simulink model "Multi_drones_final_results"  (R2021a)
settings: Solver=ode4  StartTime=0.0  StopTime=50  FixedStep=0.005  RelTol=1e-3
(part 4 of 7)

== system Multi_drones_final_results/Controller 4/Controller/Attitude controller/Sliding mode differentiator/Second-order derivative ==
  ang_d_dot : Inport
  t : Inport  Port=2
  First derivative : MATLAB Function  TreatAsAtomicUnit=on
  Memory : Memory  InitialCondition=[0;0;0]
  Memory1 : Memory
  Memory2 : Memory  InitialCondition=[0;0;0]
  ang_d_ddot : Outport
  wires:
  ang_d_dot/1 -> First derivative/1(ang_d_dot)
  First derivative/1(ang_d_ddot) -> Memory2/1
  t/1 -> First derivative/2(t)
  First derivative/3(loop_num) -> Memory1/1
  Memory1/1 -> First derivative/5("loop_num ")
  First derivative/2(ang_d_dot_prev) -> Memory/1
  Memory/1 -> First derivative/3("ang_d_dot_prev ")
  Memory2/1 -> First derivative/4("ang_d_ddot "), ang_d_ddot/1

== system Multi_drones_final_results/Controller 4/Controller/Position controller1/Position loop observer/Single Layer Neural network ==
  state : Inport
  esti_s : Inport  Port=2
  Neural network output : MATLAB Function  TreatAsAtomicUnit=on
  Update of neural weight : MATLAB Function  TreatAsAtomicUnit=on
  Weight initialisation : MATLAB Function  TreatAsAtomicUnit=on
  Weight update : Integrator  InitialConditionSource=external
  w_i : Outport
  wires:
  Update of neural weight/1(W_dot) -> Weight update/1
  esti_s/1 -> Update of neural weight/2(esti_s)
  state/1 -> Update of neural weight/1(phi_net), Neural network output/1(phi_net)
  Neural network output/1(w_i) -> w_i/1
  Weight initialisation/1(W_0) -> Weight update/2
  Weight update/1 -> Update of neural weight/3(W), Neural network output/2(W)

== system Multi_drones_final_results/Controller 5/Controller/Attitude controller/Attitude loop observer/Single Layer Neural network ==
  state : Inport
  esti_s : Inport  Port=2
  Neural network output : MATLAB Function  TreatAsAtomicUnit=on
  Update of neural weight : MATLAB Function  TreatAsAtomicUnit=on
  Weight initialisation : MATLAB Function  TreatAsAtomicUnit=on
  Weight update : Integrator  InitialConditionSource=external
  w_i : Outport
  wires:
  Update of neural weight/1(W_dot) -> Weight update/1
  esti_s/1 -> Update of neural weight/2(esti_s)
  state/1 -> Update of neural weight/1(phi_net), Neural network output/1(phi_net)
  Neural network output/1(w_i) -> w_i/1
  Weight initialisation/1(W_0) -> Weight update/2
  Weight update/1 -> Update of neural weight/3(W), Neural network output/2(W)

== system Multi_drones_final_results/Controller 5/Controller/Attitude controller/Sliding mode differentiator/First-order derivative ==
  ang_d : Inport
  t : Inport  Port=2
  First derivative : MATLAB Function  TreatAsAtomicUnit=on
  Memory : Memory  InitialCondition=[0;0;0]
  Memory1 : Memory
  Memory2 : Memory  InitialCondition=[0;0;0]
  ang_d_dot : Outport
  wires:
  ang_d/1 -> First derivative/1(ang_d)
  First derivative/1(ang_d_dot) -> Memory2/1
  t/1 -> First derivative/2(t)
  First derivative/3(loop_num) -> Memory1/1
  Memory1/1 -> First derivative/5("loop_num ")
  First derivative/2(ang_d_prev) -> Memory/1
  Memory/1 -> First derivative/3("ang_d_prev ")
  Memory2/1 -> First derivative/4("ang_d_dot "), ang_d_dot/1

== system Multi_drones_final_results/Controller 5/Controller/Attitude controller/Sliding mode differentiator/Second-order derivative ==
  ang_d_dot : Inport
  t : Inport  Port=2
  First derivative : MATLAB Function  TreatAsAtomicUnit=on
  Memory : Memory  InitialCondition=[0;0;0]
  Memory1 : Memory
  Memory2 : Memory  InitialCondition=[0;0;0]
  ang_d_ddot : Outport
  wires:
  ang_d_dot/1 -> First derivative/1(ang_d_dot)
  First derivative/1(ang_d_ddot) -> Memory2/1
  t/1 -> First derivative/2(t)
  First derivative/3(loop_num) -> Memory1/1
  Memory1/1 -> First derivative/5("loop_num ")
  First derivative/2(ang_d_dot_prev) -> Memory/1
  Memory/1 -> First derivative/3("ang_d_dot_prev ")
  Memory2/1 -> First derivative/4("ang_d_ddot "), ang_d_ddot/1

== system Multi_drones_final_results/Controller 5/Controller/Position controller1/Position loop observer/Single Layer Neural network ==
  state : Inport
  esti_s : Inport  Port=2
  Neural network output : MATLAB Function  TreatAsAtomicUnit=on
  Update of neural weight : MATLAB Function  TreatAsAtomicUnit=on
  Weight initialisation : MATLAB Function  TreatAsAtomicUnit=on
  Weight update : Integrator  InitialConditionSource=external
  w_i : Outport
  wires:
  Update of neural weight/1(W_dot) -> Weight update/1
  esti_s/1 -> Update of neural weight/2(esti_s)
  state/1 -> Update of neural weight/1(phi_net), Neural network output/1(phi_net)
  Neural network output/1(w_i) -> w_i/1
  Weight initialisation/1(W_0) -> Weight update/2
  Weight update/1 -> Update of neural weight/3(W), Neural network output/2(W)

== system Multi_drones_final_results/Controller 6/Controller/Attitude controller/Attitude loop observer/Single Layer Neural network ==
  state : Inport
  esti_s : Inport  Port=2
  Neural network output : MATLAB Function  TreatAsAtomicUnit=on
  Update of neural weight : MATLAB Function  TreatAsAtomicUnit=on
  Weight initialisation : MATLAB Function  TreatAsAtomicUnit=on
  Weight update : Integrator  InitialConditionSource=external
  w_i : Outport
  wires:
  Update of neural weight/1(W_dot) -> Weight update/1
  esti_s/1 -> Update of neural weight/2(esti_s)
  state/1 -> Update of neural weight/1(phi_net), Neural network output/1(phi_net)
  Neural network output/1(w_i) -> w_i/1
  Weight initialisation/1(W_0) -> Weight update/2
  Weight update/1 -> Update of neural weight/3(W), Neural network output/2(W)

== system Multi_drones_final_results/Controller 6/Controller/Attitude controller/Sliding mode differentiator/First-order derivative ==
  ang_d : Inport
  t : Inport  Port=2
  First derivative : MATLAB Function  TreatAsAtomicUnit=on
  Memory : Memory  InitialCondition=[0;0;0]
  Memory1 : Memory
  Memory2 : Memory  InitialCondition=[0;0;0]
  ang_d_dot : Outport
  wires:
  ang_d/1 -> First derivative/1(ang_d)
  First derivative/1(ang_d_dot) -> Memory2/1
  t/1 -> First derivative/2(t)
  First derivative/3(loop_num) -> Memory1/1
  Memory1/1 -> First derivative/5("loop_num ")
  First derivative/2(ang_d_prev) -> Memory/1
  Memory/1 -> First derivative/3("ang_d_prev ")
  Memory2/1 -> First derivative/4("ang_d_dot "), ang_d_dot/1

== system Multi_drones_final_results/Controller 6/Controller/Attitude controller/Sliding mode differentiator/Second-order derivative ==
  ang_d_dot : Inport
  t : Inport  Port=2
  First derivative : MATLAB Function  TreatAsAtomicUnit=on
  Memory : Memory  InitialCondition=[0;0;0]
  Memory1 : Memory
  Memory2 : Memory  InitialCondition=[0;0;0]
  ang_d_ddot : Outport
  wires:
  ang_d_dot/1 -> First derivative/1(ang_d_dot)
  First derivative/1(ang_d_ddot) -> Memory2/1
  t/1 -> First derivative/2(t)
  First derivative/3(loop_num) -> Memory1/1
  Memory1/1 -> First derivative/5("loop_num ")
  First derivative/2(ang_d_dot_prev) -> Memory/1
  Memory/1 -> First derivative/3("ang_d_dot_prev ")
  Memory2/1 -> First derivative/4("ang_d_ddot "), ang_d_ddot/1

== system Multi_drones_final_results/Controller 6/Controller/Position controller1/Position loop observer/Single Layer Neural network ==
  state : Inport
  esti_s : Inport  Port=2
  Neural network output : MATLAB Function  TreatAsAtomicUnit=on
  Update of neural weight : MATLAB Function  TreatAsAtomicUnit=on
  Weight initialisation : MATLAB Function  TreatAsAtomicUnit=on
  Weight update : Integrator  InitialConditionSource=external
  w_i : Outport
  wires:
  Update of neural weight/1(W_dot) -> Weight update/1
  esti_s/1 -> Update of neural weight/2(esti_s)
  state/1 -> Update of neural weight/1(phi_net), Neural network output/1(phi_net)
  Neural network output/1(w_i) -> w_i/1
  Weight initialisation/1(W_0) -> Weight update/2
  Weight update/1 -> Update of neural weight/3(W), Neural network output/2(W)

== matlab function Multi_drones_final_results/Controller 3/Controller/Position controller1/Reference selection (Low) ==
  data: ref_x_p input; x_i_p_d output; v_i_p_d output; a_i_p_d output
function [x_i_p_d, v_i_p_d, a_i_p_d] = ref_selection(ref_x_p)

%% Description
% This function is built to separate the reference states

%% Reference dividing
x_i_p_d = ref_x_p(1:3);
v_i_p_d = ref_x_p(4:6);
a_i_p_d = ref_x_p(7:9);

end

== matlab function Multi_drones_final_results/Controller 3/Controller/Position controller1/State selection ==
  data: states_i input; x_i_p output; v_i_p output
function [x_i_p, v_i_p] = state_select(states_i)

%% Description
% This is the state selection model for the self-feedback
% x_ip, v_ip, x_ia, v_ia  -> x_i, v_i
% x_ip_d, v_ip_d, a_ip_d  -> ref_x_p
% psi_i_d  -> psi_i_d (not changing)

%% System states feedback
x_i = states_i(1:6);
v_i = states_i(7:12);

x_i_p = x_i(1:3);
v_i_p = v_i(1:3);

end

== matlab function Multi_drones_final_results/Controller 3/Controller/Position controller1/Virtual position controller ==
  data: w_hat_p input; s_i_p input; delta_x_p input; delta_v_p input; a_i_p_d input; u_i_p output
function u_i_p = virtual_position_control(w_hat_p, s_i_p, delta_x_p, delta_v_p, a_i_p_d)

%% Description
% This function generates the virtual control input for the position loop
% u_i_pos = [u_ix, u_iy, u_iz] is the control input for the position loop 

%% Parameters
lambda_i_p = 2;             %% You may want to change these values
k_i_p = 3;
c_i_p = 1;

g = 9.81;                   %% Gravity constant

%% Controller design
u_i_p = a_i_p_d - w_hat_p - lambda_i_p * delta_v_p - k_i_p * delta_x_p - c_i_p * s_i_p + [0;0;g];

end

== matlab function Multi_drones_final_results/Controller 3/Controller/Real control input ==
  data: tau_i output; u_i_a input; u_i output; T_id input
function [tau_i, u_i] = real_ctr(u_i_a, T_id)

%% This function is built to obtain the actual control input (motor force)
% The functions we have are:
% T_id = u_1 + u_2 + u_3 + u_4
% u_{i,4} = (R_i/J_i_x) * (- u_2 + u_4)
% u_{i,5} = (R_i/J_i_y) * (- u_1 + u_3)
% u_{i,6} = (upsilon_i/J_i_z) * (- u_1 + u_2 - u_3 + u_4)

%% Parameter selection        
R = [0.29, 0.31, 0.30, 0.32, 0.34, 0.33] ;                  %%%%%%%%%% Change if necc

J_x = [1.25,1.23,1.24,1.23,1.24,1.25];
J_y = [1.24,1.25,1.24,1.26,1.23,1.26];
J_z = [2.50,2.52,2.51,2.49,2.50,2.53];

upsilon = [51,52,49,51,48,53]/1000;       %% Reverse moment coefficent

%% Parameter selection
serial_num = 3;         %% -- Change the serial number here

R_i = R(serial_num);

J_i_x = J_x(serial_num);
J_i_y = J_y(serial_num);
J_i_z = J_z(serial_num);

upsilon_i = upsilon(serial_num);

g_i = [ 1,1,1,1;
        0, -R_i/J_i_x, 0, R_i/J_i_x;
       -R_i/J_i_y, 0, R_i/J_i_y, 0;
       -upsilon_i/J_i_z, upsilon_i/J_i_z, -upsilon_i/J_i_z, upsilon_i/J_i_z];

u_i = g_i^(-1) * [T_id;u_i_a];

tau_1 = - u_i(2) + u_i(4);
tau_2 = - u_i(1) + u_i(3); 
tau_3 = - u_i(1) + u_i(2) - u_i(3) + u_i(4); 

tau_i = [T_id; tau_1; tau_2; tau_3];


end

== matlab function Multi_drones_final_results/Controller 1/Controller/Position controller1/Position loop observer/MATLAB Function ==
  data: t input; w_hat_p output; w_hat_p input
function w_hat_p = smooth_intro(t, w_hat_p)

% if t<=2
%     w_hat_p = zeros(3,1);
% elseif (t>2 && t<=4)
%     w_hat_p = 0.25 * (t-2)^2 * w_hat_p;
% end

eta_2 = 4;
eta_3 = 2;

f = 1 - (exp(-eta_2 * (t - eta_3))/(1 + exp(-eta_2 * (t - eta_3))) );

w_hat_p = f * w_hat_p;

end

== matlab function Multi_drones_final_results/Controller 3/Controller/Reverse calculation/Reverse calculation ==
  data: psi_i_d input; u_i_p input; atti_ref output; T_i_d output; x_i_a input
function [atti_ref, T_i_d] = reverse_calculation(psi_i_d, u_i_p, x_i_a)

%% Basic parameters of the drone   
m = [0.88,0.90,0.91,0.90,0.89,0.92] + 1.2;             %%%%%%%%%% Change if necc

serial_num = 3;
m_i = m(serial_num);
g = 9.81; 

%% Decompose information

% u_i_p = u_i_p / m_i;

u_ix = u_i_p(1);
u_iy = u_i_p(2);
u_iz = u_i_p(3);
% u_iz = u_i_p(3) + g;

phi = x_i_a(1);
theta = x_i_a(2);
psi = x_i_a(3);


%% Reverse calculation
% T_i_d = m_i * sqrt(u_ix^2 + u_iy^2 + u_iz^2);
T_i_d = m_i * u_iz/(cos(phi) * cos(theta));
% T_i_d = m_i * (u_ix * (sin(theta) * cos(psi) * cos(phi) + sin(psi) * sin(phi)) + u_iy * (sin(theta) * sin(psi) * cos(phi) - cos(psi) * sin(phi)) + u_iz * cos(theta) * cos(phi) );

phi_i_d = asin( (u_ix * sin(psi_i_d) - u_iy * cos(psi_i_d) )/sqrt(u_ix^2 + u_iy^2 + u_iz^2) );
% phi_i_d = asin( (u_ix * sin(psi_i_d) - u_iy * cos(psi_i_d) )/T_i_d );
theta_i_d = atan( (u_ix * cos(psi_i_d) + u_iy *sin(psi_i_d) )/u_iz );

% Some possible restrictions
phi_i_d = sign(phi_i_d) * min(abs(phi_i_d), pi/3);
theta_i_d = sign(theta_i_d) * min(abs(theta_i_d), pi/3);

atti_ref = [phi_i_d; theta_i_d; psi_i_d];

end

== matlab function Multi_drones_final_results/Controller 3/Controller/Reverse calculation/State selection ==
  data: states_i input; x_i_a output
function x_i_a = state_selection(states_i)

x_i_a = states_i(4:6);

end

== matlab function Multi_drones_final_results/Controller 3/High-level system/Controller ==
  data: u_i output; delta_xi input; delta_vi input; s_i input; sat_dot input; a_di input
function u_i = low_control(delta_xi, delta_vi, s_i, sat_dot, a_di)

%% This is the controller design for each agent
%% Controller parameter
c_i = 1;
lambda_i = 2;
k_i = 1.5;

%% Nominal control input
u_i = a_di - c_i * s_i - lambda_i * diag(sat_dot) * delta_vi - k_i * delta_xi;

tau_i = 0.19;
psi = 0.01;

dimension = 3;

for i = 1 : dimension
   if abs(u_i(i)) <= tau_i
       continue;
   else
       u_i(i) = sign(u_i(i)) * (tau_i + psi*exp((tau_i - abs(u_i(i)))/psi ));
   end 
end

end

== matlab function Multi_drones_final_results/Controller 3/High-level system/Information subtracting ==
  data: L input; info_commu input; bar_delta input; delta_xi output; delta_vi output; s_i output; sat_dot output
function [delta_xi, delta_vi, s_i, sat_dot]=info_subtracting(L, info_commu, bar_delta)

%% This function is built to subtract the useful information for the controller design

% info_commu is in the format of [x_1,v_1,....,x_N,v_N]
% info_control is in the format of [delta_xi, delta_vi, a_di, w_i_hat]

dimension = 3;
lambda = 2;
serial_num = 3;

L_i = L(serial_num,:);

% For multiple system test: info_commu

x_sub = kron(kron(L_i,[1,0]),eye(dimension));
v_sub = kron(kron(L_i,[0,1]),eye(dimension));

e_xi = x_sub * info_commu;
e_vi = v_sub * info_commu;

% Substracting info_control
delta_xi = bar_delta(dimension*0+1:dimension*1);
delta_vi = bar_delta(dimension*1+1:dimension*2);

% Slide variable
tau = 0.5;
phi = 0.05;

e_x_sat = zeros(size(e_xi));
sat_dot = zeros(size(e_xi));
for i = 1 : dimension
    if e_xi(i)>tau
        e_x_sat(i) = tau + phi * (1 - exp( (tau - e_xi(i))/phi ) );
        sat_dot(i) = exp( (tau - e_xi(i))/phi );
    elseif e_xi(i)<-tau
        e_x_sat(i) = - tau - phi * (1 - exp( (tau + e_xi(i))/phi ) );
        sat_dot(i) = exp( (tau + e_xi(i))/phi );
    else
        e_x_sat(i) = e_xi(i);
        sat_dot(i) = 1;
    end
end

s_i = lambda * e_x_sat + e_vi;

end

== matlab function Multi_drones_final_results/Controller 3/Quadcopter model/Quadcopter dynamics ==
  data: x_i input; u_i input; t input; x_ddot output; w_a output; w_p output; v_i input
function [x_ddot, w_a, w_p] = quad_model(x_i, u_i, t, v_i)

%% Description
% This is the function that illustrates the quadcopter dynamics
% Model from IJRNC DOI: 10.1002/rnc.5870

%% System parameters (need to be changed)
% m: quadcopter mass
% R: quadcopter radius
% c: force to moment transfer constant
% J_1: the rotation inertia around X axis
% J_2: the rotation inertia around Y axis
% J_3: the rotation inertia around Z axis
% K: aerodynamic damping coefficient
% K_F: aerodynamic friction coefficient

m = [0.88,0.90,0.91,0.90,0.89,0.92] + 1.2;             %%%%%%%%%% Change if necc
R = [0.29, 0.31, 0.30, 0.32, 0.34, 0.33] ;

J_x = [1.25,1.25,1.25,1.25,1.25,1.25];
J_y = [1.25,1.25,1.25,1.25,1.25,1.25];
J_z = [2.5,2.5,2.5,2.5,2.5,2.5];

upsilon = [5,5,5,5,5,5]/100;       %% Reverse moment coefficent

K_p = [0.012, 0.013, 0.014, 0.011, 0.012, 0.013];
K_a = [0.012, 0.013, 0.014, 0.011, 0.012, 0.013];

g = 9.81;

%% Parameter selection
serial_num = 3;         %% -- Change the serial number here

m_i = m(serial_num);
R_i = R(serial_num);

J_i_x = J_x(serial_num);
J_i_y = J_y(serial_num);
J_i_z = J_z(serial_num);

upsilon_i = upsilon(serial_num);

K_i = K_p(serial_num);
K_x = K_i;
K_y = K_i;
K_z = K_i;

K_f = K_a(serial_num);
K_phi = K_f;
K_theta = K_f;
K_psi = K_f;

%% System states selection
x_i_p = x_i(1:3);
x_i_a = x_i(4:6);

v_i_p = v_i(1:3);
v_i_a = v_i(4:6);

x = x_i_p(1);
y = x_i_p(2);
z = x_i_p(3);

phi = x_i_a(1);
theta = x_i_a(2);
psi = x_i_a(3);

v_x = v_i_p(1);
v_y = v_i_p(2);
v_z = v_i_p(3);

v_phi = v_i_a(1);
v_theta = v_i_a(2);
v_psi = v_i_a(3);

%% Control gain matrix
%% Position loop
% System dynamics
f_x = - K_x / m_i * v_x;
f_y = - K_y / m_i * v_y;
f_z = - K_z / m_i * v_z;
f_p = [f_x; f_y; f_z]; 

% Combined uncertainty
% bar_w_i_p = 0.5 * [ 0.6*sin(0.3*t + pi/5*serial_num); 0.8*sin(0.2*t + pi/5*serial_num) ; 0];
bar_w_x = 0.3 * sin(0.3*t + pi/6*serial_num);
bar_w_y = 0.4  *sin(0.2*t + pi/5*serial_num);
bar_w_z = 0.45  *sin(0.2*t + pi/4*serial_num);
bar_w_i_p = 2 * [bar_w_x; bar_w_y; bar_w_z];

w_p = f_p + bar_w_i_p ;

% Control gain matrix
g_x_1 = cos(phi) * sin(theta) * cos(psi) + sin(phi) * sin(psi);
g_x_2 = cos(phi) * sin(theta) * sin(psi) - sin(phi) * cos(psi);
g_x_3 = cos(phi) * cos(theta);
g_p = [g_x_1; g_x_2; g_x_3]/m_i;

T_i = ones(1,4) * u_i;

% T_i_d = u_i(1);

u_nom_p = g_p * T_i;

p_ddot = w_p + u_nom_p - [0;0;g];
% p_ddot = zeros(3,1);

%% Attitude loop
% System dynamics
f_phi = v_theta * v_psi * (J_i_y - J_i_z)/J_i_x - K_phi/J_i_x * v_phi;
f_theta = v_phi * v_psi * (J_i_z - J_i_x)/J_i_y - K_theta/J_i_y * v_theta;
f_psi = v_phi * v_theta * (J_i_x - J_i_y)/J_i_z - K_psi/J_i_z * v_psi;
f_i_a = [f_phi; f_theta; f_psi];

% Uncertainty
bar_w_phi = 0.05 * sin(0.5 * t - pi/6*serial_num);
bar_w_theta = 0.04 * sin(0.6 * t - pi/5*serial_num);
bar_w_psi = 0.03 * sin(0.4 * t - pi/4*serial_num);

% Combined uncertainty
bar_w_i_a = 2 * [bar_w_phi; bar_w_theta; bar_w_psi];
w_a = f_i_a + bar_w_i_a;

% Control gain matrix
g_a = [0, -R_i/J_i_x, 0, R_i/J_i_x;
       -R_i/J_i_y, 0, R_i/J_i_y, 0;
       -upsilon_i/J_i_z, upsilon_i/J_i_z, -upsilon_i/J_i_z, upsilon_i/J_i_z];

u_nom_a = g_a * u_i;   

% u_i_a = u_i(2:4);

% Acceleration
a_ddot = w_a + u_nom_a;

% States combine
x_ddot = [p_ddot; a_ddot];

% if (x_i_p(3) <= 0) && (x_ddot(3) <= 0) 
%     x_ddot(3) = 0;
% end



end

== matlab function Multi_drones_final_results/High-Level Prepare 3/Reference selection (Low) ==
  data: ref_info input; x_i_p_d output; v_i_p_d output; a_i_p_d output; psi_i_d output
function [x_i_p_d, v_i_p_d, a_i_p_d, psi_i_d] = ref_selection(ref_info)

%% Description
% This function is built to separate the reference states

%% Reference dividing
serial_num = 3;
num_agent = size(ref_info,1)/10;

ref_x = ref_info(num_agent*3*0+1 : num_agent*3*1);
ref_v = ref_info(num_agent*3*1+1 : num_agent*3*2);
ref_a = ref_info(num_agent*3*2+1 : num_agent*3*3);

ref_psi = ref_info(1+num_agent*3*3:num_agent*10);

x_i_p_d = ref_x( (serial_num-1)*3+1 : serial_num * 3);
v_i_p_d = ref_v( (serial_num-1)*3+1 : serial_num * 3);
a_i_p_d = ref_a( (serial_num-1)*3+1 : serial_num * 3);

psi_i_d = ref_psi(serial_num);

end

== matlab function Multi_drones_final_results/High-Level Prepare 3/States selection (Virtual) ==
  data: states_virtual input; x_bar_i output; v_bar_i output
function [x_bar_i, v_bar_i] = state_select_vir(states_virtual)

x_bar_i = states_virtual(1:3);
v_bar_i = states_virtual(4:6);

end

== matlab function Multi_drones_final_results/High-Level Prepare 3/Virtual error calculation ==
  data: x_bar_i input; bar_delta_x output; v_bar_i input; x_i_p_d input; v_i_p_d input; bar_delta_v output
function [bar_delta_x, bar_delta_v] = vir_error_calculation(x_bar_i, v_bar_i, x_i_p_d, v_i_p_d)

bar_delta_x = x_bar_i - x_i_p_d;
bar_delta_v = v_bar_i - v_i_p_d;

end

== matlab function Multi_drones_final_results/Controller 1/Controller/Attitude controller/Attitude loop observer/Single Layer Neural network/Neural network output ==
  data: phi_net input; w_i output; W input
function w_i = neural_output(phi_net, W)

w_i = W' * phi_net;

end

== matlab function Multi_drones_final_results/Controller 4/Controller/Attitude controller/Angle controller ==
  data: w_hat_a input; s_i_a input; delta_x_a input; delta_v_a input; u_i_a output; ang_d_ddot input
function u_i_a = angle_reference_estimator(w_hat_a, s_i_a, delta_x_a, delta_v_a, ang_d_ddot)

%% Parameters
lambda_i_a = 2;
k_i_a = 4;
c_i_a = 4;

%% Controller design
u_i_a = ang_d_ddot - w_hat_a - lambda_i_a * delta_v_a - k_i_a * delta_x_a - c_i_a * s_i_a;

end

== matlab function Multi_drones_final_results/Controller 4/Controller/Attitude controller/Angle error ==
  data: x_i_a input; v_i_a input; ang_d input; ang_d_dot input; delta_x_a output; delta_v_a output
function [delta_x_a, delta_v_a] = angle_error_calculation(x_i_a, v_i_a, ang_d, ang_d_dot)

%% This function is built to calculate the angle error
delta_x_a = x_i_a - ang_d;
delta_v_a = v_i_a - ang_d_dot;

end

== matlab function Multi_drones_final_results/Controller 4/Controller/Attitude controller/Angle sliding variable ==
  data: delta_x_a input; s_i_a output; delta_v_a input
function s_i_a = ang_slide(delta_x_a, delta_v_a)

lambda_i_a = 2;     %%%%%%%%%% Might be changed

s_i_a = delta_v_a + lambda_i_a * delta_x_a;

end

== matlab function Multi_drones_final_results/Controller 4/Controller/Attitude controller/Attitude loop observer/Error calculation ==
  data: x_i_a input; x_tilde_a output; v_i_a input; x_hat_a input; v_hat_a input; v_tilde_a output
function [x_tilde_a, v_tilde_a] = error_cal(x_i_a, v_i_a, x_hat_a, v_hat_a)

x_tilde_a = x_i_a - x_hat_a;
v_tilde_a = v_i_a - v_hat_a;

end

== matlab function Multi_drones_final_results/Controller 4/Controller/Attitude controller/Attitude loop observer/MATLAB Function ==
  data: x_tilde_a input; s_tilde_a output; v_tilde_a input
function s_tilde_a = sliding_variable(x_tilde_a, v_tilde_a)

lambda_tilde = 3;
s_tilde_a = v_tilde_a + lambda_tilde * x_tilde_a;

end

== matlab function Multi_drones_final_results/Controller 4/Controller/Attitude controller/Attitude loop observer/MATLAB Function1 ==
  data: t input; w_hat_a output; w_hat_a input
function w_hat_a = smooth_intro(t, w_hat_a)

% if t<=2
%     w_hat_a = zeros(3,1);
% elseif (t>2 && t<=4)
%     w_hat_a = 0.25 * (t-2)^2 * w_hat_a;
% end

eta_2 = 4;
eta_3 = 2;

f = 1 - (exp(-eta_2 * (t - eta_3))/(1 + exp(-eta_2 * (t - eta_3))) );

w_hat_a = f * w_hat_a;


end

== matlab function Multi_drones_final_results/Controller 4/Controller/Attitude controller/Attitude loop observer/Observation ==
  data: x_tilde_a input; u_hat_a output; v_tilde_a input; w_hat_a input; s_tilde_a input
function u_hat_a = observation(x_tilde_a, v_tilde_a, w_hat_a, s_tilde_a)

lambda_tilde = 3;
k_tilde = 2;
c_tilde = 3;

u_hat_a = w_hat_a + lambda_tilde * v_tilde_a + c_tilde * s_tilde_a + k_tilde * x_tilde_a;

end

== matlab function Multi_drones_final_results/Controller 4/Controller/Attitude controller/Attitude loop observer/Single Layer Neural network/Neural network output ==
  data: phi_net input; w_i output; W input
function w_i = neural_output(phi_net, W)

w_i = W' * phi_net;

end

== matlab function Multi_drones_final_results/Controller 4/Controller/Attitude controller/Attitude loop observer/Single Layer Neural network/Update of neural weight ==
  data: phi_net input; W_dot output; esti_s input; W input
function W_dot = weight_update(phi_net, esti_s, W)

%% This function stands for the neural weight update procedure
eta_1 = 20;
eta_2 = 0.5;

W_dot = eta_1 * phi_net * esti_s' - eta_2 * norm(esti_s) * W;

% W_dot = eta_1 * phi_net * esti_s' - eta_2 * W;

% W_dot = eta_1 * phi_net * esti_s';


end

== matlab function Multi_drones_final_results/Controller 1/Controller/Attitude controller/Angle sliding variable ==
  data: delta_x_a input; s_i_a output; delta_v_a input
function s_i_a = ang_slide(delta_x_a, delta_v_a)

lambda_i_a = 2;     %%%%%%%%%% Might be changed

s_i_a = delta_v_a + lambda_i_a * delta_x_a;

end

== matlab function Multi_drones_final_results/Controller 4/Controller/Attitude controller/Attitude loop observer/Single Layer Neural network/Weight initialisation ==
  data: W_0 output
function W_0 = weight_initial()

dimension = 6;

W_0= zeros(dimension*2,dimension/2);

end

== matlab function Multi_drones_final_results/Controller 4/Controller/Attitude controller/Attitude loop observer/Virtual system ==
  data: u_hat_a input; v_hat_dot_a output; u_nom_a input
function v_hat_dot_a = fcn(u_hat_a, u_nom_a)

v_hat_dot_a = u_nom_a + u_hat_a;

end

== matlab function Multi_drones_final_results/Controller 4/Controller/Attitude controller/Sliding mode differentiator/First-order derivative/First derivative ==
  data: ang_d input; t input; ang_d_dot output; ang_d_prev output; ang_d_prev input; ang_d_dot input; loop_num input; loop_num output
function [ang_d_dot, ang_d_prev, loop_num] = first_deri(ang_d, t, ang_d_prev, ang_d_dot, loop_num)

step = 0.005;
inter_times = 10;

if t<=step
    ang_d_dot = zeros(3,1);
else
    if t >= inter_times * loop_num * step
        ang_d_dot = (ang_d - ang_d_prev)/(step * inter_times);
        ang_d_prev = ang_d;
        loop_num = loop_num + 1;
    end
end



end

== matlab function Multi_drones_final_results/Controller 4/Controller/Attitude controller/Sliding mode differentiator/MATLAB Function ==
  data: ang_d output; z input; ang_d_dot output; ang_d_ddot output
function [ang_d, ang_d_dot, ang_d_ddot] = divide_n_send(z)

%% This function is for dividing the reference estimation for later design

dimension = 3;

ang_d = z(dimension*0+1 : dimension*1);
ang_d_dot = z(dimension*1+1 : dimension*2);
ang_d_ddot = z(dimension*2+1 : dimension*3);

end

== matlab function Multi_drones_final_results/Controller 4/Controller/Attitude controller/Sliding mode differentiator/Second-order derivative/First derivative ==
  data: ang_d_dot input; t input; ang_d_ddot output; ang_d_dot_prev output; ang_d_dot_prev input; ang_d_ddot input; loop_num input; loop_num output
function [ang_d_ddot, ang_d_dot_prev, loop_num] = second_deri(ang_d_dot, t, ang_d_dot_prev, ang_d_ddot, loop_num)

step = 0.005;
inter_times = 10;

if t<=2 * step
    ang_d_ddot = zeros(3,1);
else
    if t >= inter_times * loop_num * step
        ang_d_ddot = (ang_d_dot - ang_d_dot_prev)/(step * inter_times);
        ang_d_dot_prev = ang_d_dot;
        loop_num = loop_num + 1;
    end
end

end

== matlab function Multi_drones_final_results/Controller 4/Controller/Attitude controller/Sliding mode differentiator/sliding mode differentiator ==
  data: z input; z_dot output; x_d input
function z_dot = sliding_diff(z,x_d)

%% This is the observer function that estimates the unknown reference derivatives

dimension = 3;

alpha_1 = 8;
alpha_2 = 10;
alpha_3 = 10;
alpha_4 = 12;

beta_xd = 0.1;          %%----- Might need change

xi_1 = z(dimension*0+1:dimension*1);
xi_2 = z(dimension*1+1:dimension*2);
xi_3 = z(dimension*2+1:dimension*3);
xi_4 = z(dimension*3+1:dimension*4);

%% tunning
nu_1 = -alpha_1 * power(beta_xd,1/4) * power(abs(xi_1-x_d),3/4) .* sign(xi_1-x_d) + xi_2;
nu_2 = -alpha_2 * power(beta_xd,1/3) * power(abs(xi_2-nu_1),2/3) .* sign(xi_2-nu_1) +xi_3;
nu_3 = -alpha_3 * power(beta_xd,1/2) * power(abs(xi_3-nu_2),1/2) .* sign(xi_3-nu_2) +xi_4;
nu_4 = -alpha_4 * beta_xd .* sign(xi_4-nu_3);

z_dot = [nu_1;nu_2;nu_3;nu_4];


end

== matlab function Multi_drones_final_results/Controller 4/Controller/Attitude controller/State selection ==
  data: states_i input; x_i_a output; v_i_a output
function [x_i_a, v_i_a] = state_select(states_i)

%% This function is built to select the attitude information
% states_i = [x_i_p; x_i_a; v_i_p; v_i_a]
x_i_a = states_i(4:6);
v_i_a = states_i(10:12);

end

== matlab function Multi_drones_final_results/Controller 4/Controller/Nominal control calculation ==
  data: u_nom_p output; states_i input; u_i input; u_nom_a output
function [u_nom_p, u_nom_a] = nominal_control_cal(states_i, u_i)

%% Introduction:
% This function aims to calculate the nominal control input in different
% loop and feed them to the observers

%% System parameter
m = [0.88,0.90,0.91,0.90,0.89,0.92] + 1.2;             %%%%%%%%%% Change if necc
R = [0.29, 0.31, 0.30, 0.32, 0.34, 0.33] ;

J_x = [1.25,1.23,1.24,1.23,1.24,1.25];
J_y = [1.24,1.25,1.24,1.26,1.23,1.26];
J_z = [2.50,2.52,2.51,2.49,2.50,2.53];

upsilon = [51,52,49,51,48,53]/1000;       %% Reverse moment coefficent

%% Parameter selection
%% Parameter selection
serial_num = 4;         %% -- Change the serial number here

m_i = m(serial_num);
R_i = R(serial_num);

J_i_x = J_x(serial_num);
J_i_y = J_y(serial_num);
J_i_z = J_z(serial_num);

upsilon_i = upsilon(serial_num);

%% System states
x_i_a = states_i(4:6);

phi = x_i_a(1);
theta = x_i_a(2);
psi = x_i_a(3);

%% Control gain matrix
% Position loop
g_x_1 = cos(phi) * sin(theta) * cos(psi) + sin(phi) * sin(psi);
g_x_2 = cos(phi) * sin(theta) * sin(psi) - sin(phi) * cos(psi);
g_x_3 = cos(phi) * cos(theta);
g_p = [g_x_1; g_x_2; g_x_3]/m_i;

% Attitude loop
g_a = [0, -R_i/J_i_x, 0, R_i/J_i_x;
       -R_i/J_i_y, 0, R_i/J_i_y, 0;
       -upsilon_i/J_i_z, upsilon_i/J_i_z, -upsilon_i/J_i_z, upsilon_i/J_i_z];

%% Nominal control input
u_nom_p = g_p * ([1,1,1,1] * u_i);

u_nom_a = g_a * u_i;


end

== matlab function Multi_drones_final_results/Controller 1/Controller/Real control input ==
  data: tau_i output; u_i_a input; u_i output; T_id input
function [tau_i, u_i] = real_ctr(u_i_a, T_id)

%% This function is built to obtain the actual control input (motor force)
% The functions we have are:
% T_id = u_1 + u_2 + u_3 + u_4
% u_{i,4} = (R_i/J_i_x) * (- u_2 + u_4)
% u_{i,5} = (R_i/J_i_y) * (- u_1 + u_3)
% u_{i,6} = (upsilon_i/J_i_z) * (- u_1 + u_2 - u_3 + u_4)

%% Parameter selection        
R = [0.29, 0.31, 0.30, 0.32, 0.34, 0.33] ;                  %%%%%%%%%% Change if necc

J_x = [1.25,1.23,1.24,1.23,1.24,1.25];
J_y = [1.24,1.25,1.24,1.26,1.23,1.26];
J_z = [2.50,2.52,2.51,2.49,2.50,2.53];

upsilon = [51,52,49,51,48,53]/1000;       %% Reverse moment coefficent

%% Parameter selection
serial_num = 1;         %% -- Change the serial number here

R_i = R(serial_num);

J_i_x = J_x(serial_num);
J_i_y = J_y(serial_num);
J_i_z = J_z(serial_num);

upsilon_i = upsilon(serial_num);

g_i = [ 1,1,1,1;
        0, -R_i/J_i_x, 0, R_i/J_i_x;
       -R_i/J_i_y, 0, R_i/J_i_y, 0;
       -upsilon_i/J_i_z, upsilon_i/J_i_z, -upsilon_i/J_i_z, upsilon_i/J_i_z];

u_i = g_i^(-1) * [T_id;u_i_a];

tau_1 = - u_i(2) + u_i(4);
tau_2 = - u_i(1) + u_i(3); 
tau_3 = - u_i(1) + u_i(2) - u_i(3) + u_i(4); 

tau_i = [T_id; tau_1; tau_2; tau_3];


end

== matlab function Multi_drones_final_results/Controller 4/Controller/Position controller1/Error calculation ==
  data: s_i_p output; x_i_p input; delta_x_p output; v_i_p input; Phi_i input; x_i_p_d input; v_i_p_d input; delta_v_p output
function [s_i_p, delta_x_p, delta_v_p] = error_cal(x_i_p, v_i_p, Phi_i, x_i_p_d, v_i_p_d)

%% Description
% This function is built to calculate the tracking errors and the sliding variable

%% Error states calculation
delta_x_p = x_i_p - x_i_p_d;
delta_v_p = v_i_p - v_i_p_d;

%% Sliding variable calculation
lambda_p = 2;           %% You may want to change this

s_i_p = delta_v_p + lambda_p * (delta_x_p - Phi_i);

end

== matlab function Multi_drones_final_results/Controller 4/Controller/Position controller1/Position loop observer/Error calculation ==
  data: x_i_p input; x_tilde_p output; v_i_p input; x_hat_p input; v_hat_p input; v_tilde_p output
function [x_tilde_p, v_tilde_p] = error_cal(x_i_p, v_i_p, x_hat_p, v_hat_p)

%% Description
% This function calculates the tracking error for the observer states

x_tilde_p = x_i_p - x_hat_p;
v_tilde_p = v_i_p - v_hat_p;

end

== matlab function Multi_drones_final_results/Controller 4/Controller/Position controller1/Position loop observer/MATLAB Function ==
  data: t input; w_hat_p output; w_hat_p input
function w_hat_p = smooth_intro(t, w_hat_p)

% if t<=2
%     w_hat_p = zeros(3,1);
% elseif (t>2 && t<=4)
%     w_hat_p = 0.25 * (t-2)^2 * w_hat_p;
% end

eta_2 = 4;
eta_3 = 2;

f = 1 - (exp(-eta_2 * (t - eta_3))/(1 + exp(-eta_2 * (t - eta_3))) );

w_hat_p = f * w_hat_p;

end

== matlab function Multi_drones_final_results/Controller 4/Controller/Position controller1/Position loop observer/Observation ==
  data: x_tilde_p input; u_hat_p output; v_tilde_p input; w_hat_p input; s_tilde_p input
function u_hat_p = observation(x_tilde_p, v_tilde_p, w_hat_p, s_tilde_p)

%% Description
% This function calculates the observation for position loop

%% Controller parameters
lambda_tilde = 2;           %% You may want to change that 
k_tilde = 4;
c_tilde = 4;

%% Final observation
u_hat_p = w_hat_p + lambda_tilde * v_tilde_p + c_tilde * s_tilde_p + k_tilde * x_tilde_p;

end

== matlab function Multi_drones_final_results/Controller 4/Controller/Position controller1/Position loop observer/Single Layer Neural network/Neural network output ==
  data: phi_net input; w_i output; W input
function w_i = neural_output(phi_net, W)

w_i = W' * phi_net;

end

== matlab function Multi_drones_final_results/Controller 4/Controller/Position controller1/Position loop observer/Single Layer Neural network/Update of neural weight ==
  data: phi_net input; W_dot output; esti_s input; W input
function W_dot = weight_update(phi_net, esti_s, W)

%% This function stands for the neural weight update procedure
eta_1 = 20;
eta_2 = 0.5;

W_dot = eta_1 * phi_net * esti_s' - eta_2 * norm(esti_s) * W;

% W_dot = eta_1 * phi_net * esti_s' - eta_2 * W;

% W_dot = eta_1 * phi_net * esti_s';


end

== matlab function Multi_drones_final_results/Controller 4/Controller/Position controller1/Position loop observer/Single Layer Neural network/Weight initialisation ==
  data: W_0 output
function W_0 = weight_initial()

dimension = 6;

W_0= zeros(dimension*2,dimension/2);

end

== matlab function Multi_drones_final_results/Controller 4/Controller/Position controller1/Position loop observer/Sliding variable calculation ==
  data: x_tilde_p input; s_tilde_p output; v_tilde_p input
function s_tilde_p = sliding_variable(x_tilde_p, v_tilde_p)

%% Description
% This function calculates the observation sliding surface

lambda_tilde = 2;           %% You may need to change the value
s_tilde_p = v_tilde_p + lambda_tilde * x_tilde_p;

end

== matlab function Multi_drones_final_results/Controller 4/Controller/Position controller1/Position loop observer/Virtual system ==
  data: u_hat_p input; v_hat_dot_p output; u_nom_p input
function v_hat_dot_p = fcn(u_hat_p, u_nom_p)

%% Description
% This function updates the states in the observer

%% Gravity constant
g = 9.81;

%% State update
v_hat_dot_p = u_nom_p + u_hat_p - [0;0;g];

end

== matlab function Multi_drones_final_results/Controller 4/Controller/Position controller1/Reference selection (Low) ==
  data: ref_x_p input; x_i_p_d output; v_i_p_d output; a_i_p_d output
function [x_i_p_d, v_i_p_d, a_i_p_d] = ref_selection(ref_x_p)

%% Description
% This function is built to separate the reference states

%% Reference dividing
x_i_p_d = ref_x_p(1:3);
v_i_p_d = ref_x_p(4:6);
a_i_p_d = ref_x_p(7:9);

end

== matlab function Multi_drones_final_results/Controller 1/Controller/Attitude controller/Attitude loop observer/Single Layer Neural network/Update of neural weight ==
  data: phi_net input; W_dot output; esti_s input; W input
function W_dot = weight_update(phi_net, esti_s, W)

%% This function stands for the neural weight update procedure
eta_1 = 20;
eta_2 = 0.5;

W_dot = eta_1 * phi_net * esti_s' - eta_2 * norm(esti_s) * W;

% W_dot = eta_1 * phi_net * esti_s' - eta_2 * W;

% W_dot = eta_1 * phi_net * esti_s';


end

== matlab function Multi_drones_final_results/Controller 4/Controller/Position controller1/State selection ==
  data: states_i input; x_i_p output; v_i_p output
function [x_i_p, v_i_p] = state_select(states_i)

%% Description
% This is the state selection model for the self-feedback
% x_ip, v_ip, x_ia, v_ia  -> x_i, v_i
% x_ip_d, v_ip_d, a_ip_d  -> ref_x_p
% psi_i_d  -> psi_i_d (not changing)

%% System states feedback
x_i = states_i(1:6);
v_i = states_i(7:12);

x_i_p = x_i(1:3);
v_i_p = v_i(1:3);

end

== matlab function Multi_drones_final_results/Controller 4/Controller/Position controller1/Virtual position controller ==
  data: w_hat_p input; s_i_p input; delta_x_p input; delta_v_p input; a_i_p_d input; u_i_p output
function u_i_p = virtual_position_control(w_hat_p, s_i_p, delta_x_p, delta_v_p, a_i_p_d)

%% Description
% This function generates the virtual control input for the position loop
% u_i_pos = [u_ix, u_iy, u_iz] is the control input for the position loop 

%% Parameters
lambda_i_p = 2;             %% You may want to change these values
k_i_p = 3;
c_i_p = 1;

g = 9.81;                   %% Gravity constant

%% Controller design
u_i_p = a_i_p_d - w_hat_p - lambda_i_p * delta_v_p - k_i_p * delta_x_p - c_i_p * s_i_p + [0;0;g];

end

== matlab function Multi_drones_final_results/Controller 4/Controller/Real control input ==
  data: tau_i output; u_i_a input; u_i output; T_id input
function [tau_i, u_i] = real_ctr(u_i_a, T_id)

%% This function is built to obtain the actual control input (motor force)
% The functions we have are:
% T_id = u_1 + u_2 + u_3 + u_4
% u_{i,4} = (R_i/J_i_x) * (- u_2 + u_4)
% u_{i,5} = (R_i/J_i_y) * (- u_1 + u_3)
% u_{i,6} = (upsilon_i/J_i_z) * (- u_1 + u_2 - u_3 + u_4)

%% Parameter selection        
R = [0.29, 0.31, 0.30, 0.32, 0.34, 0.33] ;                  %%%%%%%%%% Change if necc

J_x = [1.25,1.23,1.24,1.23,1.24,1.25];
J_y = [1.24,1.25,1.24,1.26,1.23,1.26];
J_z = [2.50,2.52,2.51,2.49,2.50,2.53];

upsilon = [51,52,49,51,48,53]/1000;       %% Reverse moment coefficent

%% Parameter selection
serial_num = 4;         %% -- Change the serial number here

R_i = R(serial_num);

J_i_x = J_x(serial_num);
J_i_y = J_y(serial_num);
J_i_z = J_z(serial_num);

upsilon_i = upsilon(serial_num);

g_i = [ 1,1,1,1;
        0, -R_i/J_i_x, 0, R_i/J_i_x;
       -R_i/J_i_y, 0, R_i/J_i_y, 0;
       -upsilon_i/J_i_z, upsilon_i/J_i_z, -upsilon_i/J_i_z, upsilon_i/J_i_z];

u_i = g_i^(-1) * [T_id;u_i_a];

tau_1 = - u_i(2) + u_i(4);
tau_2 = - u_i(1) + u_i(3); 
tau_3 = - u_i(1) + u_i(2) - u_i(3) + u_i(4); 

tau_i = [T_id; tau_1; tau_2; tau_3];


end

== matlab function Multi_drones_final_results/Controller 4/Controller/Reverse calculation/Reverse calculation ==
  data: psi_i_d input; u_i_p input; atti_ref output; T_i_d output; x_i_a input
function [atti_ref, T_i_d] = reverse_calculation(psi_i_d, u_i_p, x_i_a)

%% Basic parameters of the drone   
m = [0.88,0.90,0.91,0.90,0.89,0.92] + 1.2;             %%%%%%%%%% Change if necc

serial_num = 4;
m_i = m(serial_num);
g = 9.81;

%% Decompose information

% u_i_p = u_i_p / m_i;

u_ix = u_i_p(1);
u_iy = u_i_p(2);
u_iz = u_i_p(3);
% u_iz = u_i_p(3) + g;

phi = x_i_a(1);
theta = x_i_a(2);
psi = x_i_a(3);


%% Reverse calculation
% T_i_d = m_i * sqrt(u_ix^2 + u_iy^2 + u_iz^2);
T_i_d = m_i * u_iz/(cos(phi) * cos(theta));
% T_i_d = m_i * (u_ix * (sin(theta) * cos(psi) * cos(phi) + sin(psi) * sin(phi)) + u_iy * (sin(theta) * sin(psi) * cos(phi) - cos(psi) * sin(phi)) + u_iz * cos(theta) * cos(phi) );

phi_i_d = asin( (u_ix * sin(psi_i_d) - u_iy * cos(psi_i_d) )/sqrt(u_ix^2 + u_iy^2 + u_iz^2) );
% phi_i_d = asin( (u_ix * sin(psi_i_d) - u_iy * cos(psi_i_d) )/T_i_d );
theta_i_d = atan( (u_ix * cos(psi_i_d) + u_iy *sin(psi_i_d) )/u_iz );

% Some possible restrictions
phi_i_d = sign(phi_i_d) * min(abs(phi_i_d), pi/3);
theta_i_d = sign(theta_i_d) * min(abs(theta_i_d), pi/3);

atti_ref = [phi_i_d; theta_i_d; psi_i_d];

end

== matlab function Multi_drones_final_results/Controller 4/Controller/Reverse calculation/State selection ==
  data: states_i input; x_i_a output
function x_i_a = state_selection(states_i)

x_i_a = states_i(4:6);

end

== matlab function Multi_drones_final_results/Controller 4/High-level system/Controller ==
  data: u_i output; delta_xi input; delta_vi input; s_i input; sat_dot input; a_di input
function u_i = low_control(delta_xi, delta_vi, s_i, sat_dot, a_di)

%% This is the controller design for each agent
%% Controller parameter
c_i = 1;
lambda_i = 2;
k_i = 1.5;

%% Nominal control input
u_i = a_di - c_i * s_i - lambda_i * diag(sat_dot) * delta_vi - k_i * delta_xi;

tau_i = 0.19;
psi = 0.01;

dimension = 3;

for i = 1 : dimension
   if abs(u_i(i)) <= tau_i
       continue;
   else
       u_i(i) = sign(u_i(i)) * (tau_i + psi*exp((tau_i - abs(u_i(i)))/psi ));
   end 
end

end

== matlab function Multi_drones_final_results/Controller 4/High-level system/Information subtracting ==
  data: L input; info_commu input; bar_delta input; delta_xi output; delta_vi output; s_i output; sat_dot output
function [delta_xi, delta_vi, s_i, sat_dot]=info_subtracting(L, info_commu, bar_delta)

%% This function is built to subtract the useful information for the controller design

% info_commu is in the format of [x_1,v_1,....,x_N,v_N]
% info_control is in the format of [delta_xi, delta_vi, a_di, w_i_hat]

dimension = 3;
lambda = 2;
serial_num = 4;

L_i = L(serial_num,:);

% For multiple system test: info_commu

x_sub = kron(kron(L_i,[1,0]),eye(dimension));
v_sub = kron(kron(L_i,[0,1]),eye(dimension));

e_xi = x_sub * info_commu;
e_vi = v_sub * info_commu;

% Substracting info_control
delta_xi = bar_delta(dimension*0+1:dimension*1);
delta_vi = bar_delta(dimension*1+1:dimension*2);

% Slide variable
tau = 0.5;
phi = 0.05;

e_x_sat = zeros(size(e_xi));
sat_dot = zeros(size(e_xi));
for i = 1 : dimension
    if e_xi(i)>tau
        e_x_sat(i) = tau + phi * (1 - exp( (tau - e_xi(i))/phi ) );
        sat_dot(i) = exp( (tau - e_xi(i))/phi );
    elseif e_xi(i)<-tau
        e_x_sat(i) = - tau - phi * (1 - exp( (tau + e_xi(i))/phi ) );
        sat_dot(i) = exp( (tau + e_xi(i))/phi );
    else
        e_x_sat(i) = e_xi(i);
        sat_dot(i) = 1;
    end
end

s_i = lambda * e_x_sat + e_vi;

end

== matlab function Multi_drones_final_results/Controller 4/Quadcopter model/Quadcopter dynamics ==
  data: x_i input; u_i input; t input; x_ddot output; w_a output; w_p output; v_i input
function [x_ddot, w_a, w_p] = quad_model(x_i, u_i, t, v_i)

%% Description
% This is the function that illustrates the quadcopter dynamics
% Model from IJRNC DOI: 10.1002/rnc.5870

%% System parameters (need to be changed)
% m: quadcopter mass
% R: quadcopter radius
% c: force to moment transfer constant
% J_1: the rotation inertia around X axis
% J_2: the rotation inertia around Y axis
% J_3: the rotation inertia around Z axis
% K: aerodynamic damping coefficient
% K_F: aerodynamic friction coefficient

m = [0.88,0.90,0.91,0.90,0.89,0.92] + 1.2;             %%%%%%%%%% Change if necc
R = [0.29, 0.31, 0.30, 0.32, 0.34, 0.33] ;

J_x = [1.25,1.23,1.24,1.23,1.24,1.25];
J_y = [1.24,1.25,1.24,1.26,1.23,1.26];
J_z = [2.50,2.52,2.51,2.49,2.50,2.53];

upsilon = [51,52,49,51,48,53]/1000;       %% Reverse moment coefficent

K_p = [0.012, 0.013, 0.014, 0.011, 0.012, 0.013];
K_a = [0.012, 0.013, 0.014, 0.011, 0.012, 0.013];

g = 9.81;

%% Parameter selection
serial_num = 4;         %% -- Change the serial number here

m_i = m(serial_num);
R_i = R(serial_num);

J_i_x = J_x(serial_num);
J_i_y = J_y(serial_num);
J_i_z = J_z(serial_num);

upsilon_i = upsilon(serial_num);

K_i = K_p(serial_num);
K_x = K_i;
K_y = K_i;
K_z = K_i;

K_f = K_a(serial_num);
K_phi = K_f;
K_theta = K_f;
K_psi = K_f;

%% System states selection
x_i_p = x_i(1:3);
x_i_a = x_i(4:6);

v_i_p = v_i(1:3);
v_i_a = v_i(4:6);

x = x_i_p(1);
y = x_i_p(2);
z = x_i_p(3);

phi = x_i_a(1);
theta = x_i_a(2);
psi = x_i_a(3);

v_x = v_i_p(1);
v_y = v_i_p(2);
v_z = v_i_p(3);

v_phi = v_i_a(1);
v_theta = v_i_a(2);
v_psi = v_i_a(3);

%% Control gain matrix
%% Position loop
% System dynamics
f_x = - K_x / m_i * v_x;
f_y = - K_y / m_i * v_y;
f_z = - K_z / m_i * v_z;
f_p = [f_x; f_y; f_z]; 

% Combined uncertainty
% bar_w_i_p = 0.5 * [ 0.6*sin(0.3*t + pi/5*serial_num); 0.8*sin(0.2*t + pi/5*serial_num) ; 0];
bar_w_x = 0.3 * sin(0.3*t + pi/6*serial_num);
bar_w_y = 0.4  *sin(0.2*t + pi/5*serial_num);
bar_w_z = 0.45  *sin(0.2*t + pi/4*serial_num);
bar_w_i_p = 2 * [bar_w_x; bar_w_y; bar_w_z];

w_p = f_p + bar_w_i_p ;

% Control gain matrix
g_x_1 = cos(phi) * sin(theta) * cos(psi) + sin(phi) * sin(psi);
g_x_2 = cos(phi) * sin(theta) * sin(psi) - sin(phi) * cos(psi);
g_x_3 = cos(phi) * cos(theta);
g_p = [g_x_1; g_x_2; g_x_3]/m_i;

T_i = ones(1,4) * u_i;

% T_i_d = u_i(1);

u_nom_p = g_p * T_i;

p_ddot = w_p + u_nom_p - [0;0;g];
% p_ddot = zeros(3,1);

%% Attitude loop
% System dynamics
f_phi = v_theta * v_psi * (J_i_y - J_i_z)/J_i_x - K_phi/J_i_x * v_phi;
f_theta = v_phi * v_psi * (J_i_z - J_i_x)/J_i_y - K_theta/J_i_y * v_theta;
f_psi = v_phi * v_theta * (J_i_x - J_i_y)/J_i_z - K_psi/J_i_z * v_psi;
f_i_a = [f_phi; f_theta; f_psi];

% Uncertainty
bar_w_phi = 0.05 * sin(0.5 * t - pi/6*serial_num);
bar_w_theta = 0.04 * sin(0.6 * t - pi/5*serial_num);
bar_w_psi = 0.03 * sin(0.4 * t - pi/4*serial_num);

% Combined uncertainty
bar_w_i_a = 2 * [bar_w_phi; bar_w_theta; bar_w_psi];
w_a = f_i_a + bar_w_i_a;

% Control gain matrix
g_a = [0, -R_i/J_i_x, 0, R_i/J_i_x;
       -R_i/J_i_y, 0, R_i/J_i_y, 0;
       -upsilon_i/J_i_z, upsilon_i/J_i_z, -upsilon_i/J_i_z, upsilon_i/J_i_z];

u_nom_a = g_a * u_i;   

% u_i_a = u_i(2:4);

% Acceleration
a_ddot = w_a + u_nom_a;

% States combine
x_ddot = [p_ddot; a_ddot];

% if (x_i_p(3) <= 0) && (x_ddot(3) <= 0) 
%     x_ddot(3) = 0;
% end



end

== matlab function Multi_drones_final_results/High-Level Prepare 4/Reference selection (Low) ==
  data: ref_info input; x_i_p_d output; v_i_p_d output; a_i_p_d output; psi_i_d output
function [x_i_p_d, v_i_p_d, a_i_p_d, psi_i_d] = ref_selection(ref_info)

%% Description
% This function is built to separate the reference states

%% Reference dividing
serial_num = 4;
num_agent = size(ref_info,1)/10;

ref_x = ref_info(num_agent*3*0+1 : num_agent*3*1);
ref_v = ref_info(num_agent*3*1+1 : num_agent*3*2);
ref_a = ref_info(num_agent*3*2+1 : num_agent*3*3);

ref_psi = ref_info(1+num_agent*3*3:num_agent*10);

x_i_p_d = ref_x( (serial_num-1)*3+1 : serial_num * 3);
v_i_p_d = ref_v( (serial_num-1)*3+1 : serial_num * 3);
a_i_p_d = ref_a( (serial_num-1)*3+1 : serial_num * 3);

psi_i_d = ref_psi(serial_num);

end

== matlab function Multi_drones_final_results/Controller 1/Controller/Position controller1/Position loop observer/Observation ==
  data: x_tilde_p input; u_hat_p output; v_tilde_p input; w_hat_p input; s_tilde_p input
function u_hat_p = observation(x_tilde_p, v_tilde_p, w_hat_p, s_tilde_p)

%% Description
% This function calculates the observation for position loop

%% Controller parameters
lambda_tilde = 2;           %% You may want to change that 
k_tilde = 4;
c_tilde = 4;

%% Final observation
u_hat_p = w_hat_p + lambda_tilde * v_tilde_p + c_tilde * s_tilde_p + k_tilde * x_tilde_p;

end

== matlab function Multi_drones_final_results/High-Level Prepare 4/States selection (Virtual) ==
  data: states_virtual input; x_bar_i output; v_bar_i output
function [x_bar_i, v_bar_i] = state_select_vir(states_virtual)

x_bar_i = states_virtual(1:3);
v_bar_i = states_virtual(4:6);

end

== matlab function Multi_drones_final_results/High-Level Prepare 4/Virtual error calculation ==
  data: x_bar_i input; bar_delta_x output; v_bar_i input; x_i_p_d input; v_i_p_d input; bar_delta_v output
function [bar_delta_x, bar_delta_v] = vir_error_calculation(x_bar_i, v_bar_i, x_i_p_d, v_i_p_d)

bar_delta_x = x_bar_i - x_i_p_d;
bar_delta_v = v_bar_i - v_i_p_d;

end

== matlab function Multi_drones_final_results/Controller 5/Controller/Attitude controller/Angle controller ==
  data: w_hat_a input; s_i_a input; delta_x_a input; delta_v_a input; u_i_a output; ang_d_ddot input
function u_i_a = angle_reference_estimator(w_hat_a, s_i_a, delta_x_a, delta_v_a, ang_d_ddot)

%% Parameters
lambda_i_a = 2;
k_i_a = 4;
c_i_a = 4;

%% Controller design
u_i_a = ang_d_ddot - w_hat_a - lambda_i_a * delta_v_a - k_i_a * delta_x_a - c_i_a * s_i_a;

end

== matlab function Multi_drones_final_results/Controller 5/Controller/Attitude controller/Angle error ==
  data: x_i_a input; v_i_a input; ang_d input; ang_d_dot input; delta_x_a output; delta_v_a output
function [delta_x_a, delta_v_a] = angle_error_calculation(x_i_a, v_i_a, ang_d, ang_d_dot)

%% This function is built to calculate the angle error
delta_x_a = x_i_a - ang_d;
delta_v_a = v_i_a - ang_d_dot;

end

== matlab function Multi_drones_final_results/Controller 5/Controller/Attitude controller/Angle sliding variable ==
  data: delta_x_a input; s_i_a output; delta_v_a input
function s_i_a = ang_slide(delta_x_a, delta_v_a)

lambda_i_a = 2;     %%%%%%%%%% Might be changed

s_i_a = delta_v_a + lambda_i_a * delta_x_a;

end

== matlab function Multi_drones_final_results/Controller 5/Controller/Attitude controller/Attitude loop observer/Error calculation ==
  data: x_i_a input; x_tilde_a output; v_i_a input; x_hat_a input; v_hat_a input; v_tilde_a output
function [x_tilde_a, v_tilde_a] = error_cal(x_i_a, v_i_a, x_hat_a, v_hat_a)

x_tilde_a = x_i_a - x_hat_a;
v_tilde_a = v_i_a - v_hat_a;

end

== matlab function Multi_drones_final_results/Controller 5/Controller/Attitude controller/Attitude loop observer/MATLAB Function ==
  data: x_tilde_a input; s_tilde_a output; v_tilde_a input
function s_tilde_a = sliding_variable(x_tilde_a, v_tilde_a)

lambda_tilde = 3;
s_tilde_a = v_tilde_a + lambda_tilde * x_tilde_a;

end
